simulink model "RPEM"  (Simulink 5.0)
settings: Solver=ode45  StartTime=0.0  StopTime=100.0  RelTol=1e-3
undefined symbols (not defined in the file): ts
libraries: dspmtrx3 x6, simulink x4, dspinverses x1
settings Model: LastModifiedBy=LeO

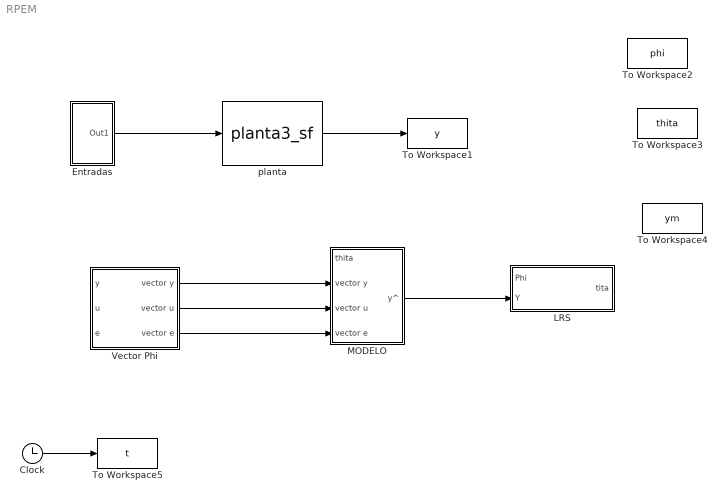
== system RPEM ==
  Clock : Clock
      settings: Decimation=10
  Entradas : Subsystem
  LRS : Subsystem
  MODELO : Subsystem
  To Workspace1 : ToWorkspace  VariableName=y  SampleTime=ts  SaveFormat=Array
  To Workspace2 : ToWorkspace  VariableName=phi  SampleTime=ts  SaveFormat=Array
  To Workspace3 : ToWorkspace  VariableName=thita  SampleTime=ts  SaveFormat=Array
  To Workspace4 : ToWorkspace  VariableName=ym  SampleTime=ts  SaveFormat=Array
  To Workspace5 : ToWorkspace  VariableName=t  SampleTime=ts  SaveFormat=Array
  Vector Phi : Subsystem  mask{nu=1, ny=3, ne=1, nk=1}
      mask prompts: nu "Nº de u tomadas"; ny "Nº de y tomadas"; ne "Nº de e tomadas"; nk "Nº de retardo"
  planta : S-Function  FunctionName=planta3_sf
  wires:
  Entradas/1(Out1) -> planta/1
  planta/1 -> To Workspace1/1
  Clock/1 -> To Workspace5/1
  MODELO/1(y^) -> LRS/2(Y)
  Vector Phi/1(vector y) -> MODELO/2(vector y)
  Vector Phi/2(vector u) -> MODELO/3(vector u)
  Vector Phi/3(vector e) -> MODELO/4("vector e ")

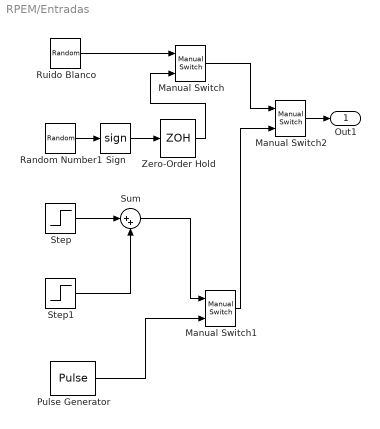
== system RPEM/Entradas ==
  Manual Switch : simulink/Signal Routing/Manual Switch  sw=0  action=0
  Manual Switch1 : simulink/Signal Routing/Manual Switch  sw=1  action=0
  Manual Switch2 : simulink/Signal Routing/Manual Switch  sw=0  action=0
  Pulse Generator : DiscretePulseGenerator  PulseType=Time based  PulseWidth=50
  Random Number1 : RandomNumber  SampleTime=0
  Ruido Blanco : RandomNumber  Variance=20  Seed=12  SampleTime=ts
  Sign : Signum
  Step : Step  Time=10  After=25  SampleTime=0.05
  Step1 : Step  Time=30  After=3  SampleTime=0.05
  Sum : Sum  Inputs=|++  SaturateOnIntegerOverflow=on
  Zero-Order Hold : ZeroOrderHold  SampleTime=0.05
  Out1 : Outport
  wires:
  Sign/1 -> Zero-Order Hold/1
  Random Number1/1 -> Sign/1
  Manual Switch/1 -> Manual Switch2/1
  Ruido Blanco/1 -> Manual Switch/1
  Zero-Order Hold/1 -> Manual Switch/2
  Manual Switch2/1 -> Out1/1
  Step/1 -> Sum/1
  Step1/1 -> Sum/2
  Manual Switch1/1 -> Manual Switch2/2
  Sum/1 -> Manual Switch1/1
  Pulse Generator/1 -> Manual Switch1/2

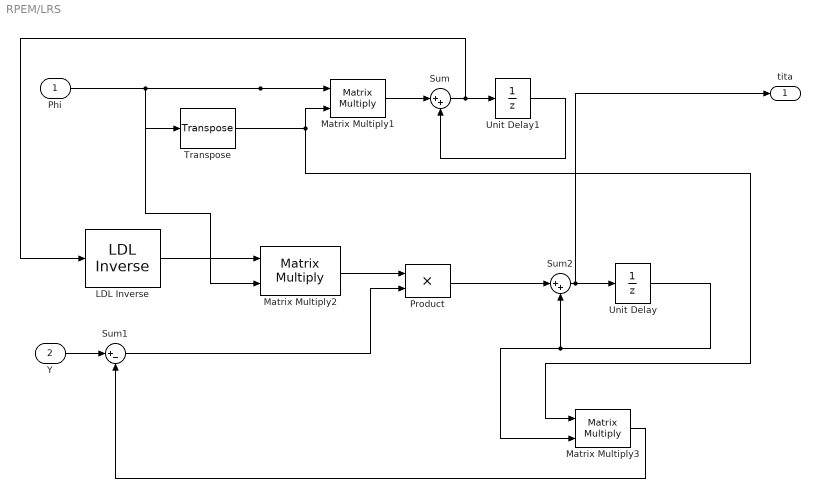
== system RPEM/LRS ==
  "Phi " : Inport  SampleTime=ts
  Y : Inport  Port=2  SampleTime=ts
  LDL Inverse : dspinverses/LDL Inverse  errmode=Ignore
  Matrix Multiply1 : dspmtrx3/Matrix Multiply  numInputPorts=2  OptimizationLevel=None
  Matrix Multiply2 : dspmtrx3/Matrix Multiply  numInputPorts=2  OptimizationLevel=None
  Matrix Multiply3 : dspmtrx3/Matrix Multiply  numInputPorts=2  OptimizationLevel=None
  Product : Product  SaturateOnIntegerOverflow=on
  Sum : Sum  Inputs=|++  SaturateOnIntegerOverflow=on
  Sum1 : Sum  Inputs=|+-  SaturateOnIntegerOverflow=on
  Sum2 : Sum  Inputs=|++  SaturateOnIntegerOverflow=on
  Transpose : dspmtrx3/Transpose  Hermitian=off
  Unit Delay : UnitDelay  X0=1*10^-3  SampleTime=ts
  Unit Delay1 : UnitDelay  X0=10^-3  SampleTime=ts
  tita : Outport
  wires:
  "Phi "/1 -> Transpose/1, Matrix Multiply2/2, Matrix Multiply1/1
  Transpose/1 -> Matrix Multiply3/1, Matrix Multiply1/2
  Matrix Multiply1/1 -> Sum/1
  Sum/1 -> Unit Delay1/1, LDL Inverse/1
  Unit Delay1/1 -> Sum/2
  LDL Inverse/1 -> Matrix Multiply2/1
  Sum2/1 -> Unit Delay/1, tita/1
  Y/1 -> Sum1/1
  Matrix Multiply2/1 -> Product/1
  Product/1 -> Sum2/1
  Matrix Multiply3/1 -> Sum1/2
  Sum1/1 -> Product/2
  Unit Delay/1 -> Matrix Multiply3/2, Sum2/2

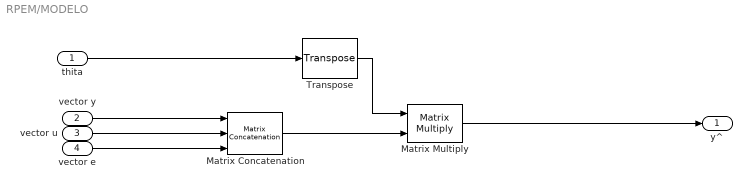
== system RPEM/MODELO ==
  thita : Inport
  vector y : Inport  Port=2
  vector u : Inport  Port=3
  "vector e " : Inport  Port=4
  Matrix Concatenation : simulink/Math Operations/Matrix Concatenation  numInports=3  catMethod=Vertical
  Matrix Multiply : dspmtrx3/Matrix Multiply  numInputPorts=2  OptimizationLevel=None
  Transpose : dspmtrx3/Transpose  Hermitian=off
  y^ : Outport
  wires:
  Matrix Concatenation/1 -> Matrix Multiply/2
  Transpose/1 -> Matrix Multiply/1
  thita/1 -> Transpose/1
  Matrix Multiply/1 -> y^/1
  "vector e "/1 -> Matrix Concatenation/3
  vector u/1 -> Matrix Concatenation/2
  vector y/1 -> Matrix Concatenation/1

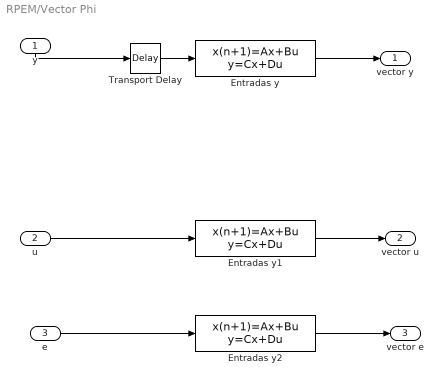
== system RPEM/Vector Phi ==
  "y " : Inport  Orientation=down  SampleTime=ts
  u : Inport  Port=2  SampleTime=ts
  e : Inport  Port=3  SampleTime=ts
  Entradas y : DiscreteStateSpace  A=[zeros(1,ny) ;eye(ny-1,ny)]  B=[[-1 zeros(1,ny-1)]']  C=[eye(ny)]  D=[zeros(1,ny)']  SampleTime=ts
  Entradas y1 : DiscreteStateSpace  A=[zeros(1,nu) ;eye(nu-1,nu)]  B=[[-1 zeros(1,nu-1)]']  C=[eye(nu)]  D=[zeros(1,nu)']  SampleTime=ts
  Entradas y2 : DiscreteStateSpace  A=[zeros(1,ne) ;eye(nu-1,ne)]  B=[[-1 zeros(1,ne-1)]']  C=[eye(ne)]  D=[zeros(1,ne)']  SampleTime=ts
  Transport Delay : TransportDelay  DelayTime=nk*ts
  vector y : Outport
  vector u : Outport  Port=2
  vector e : Outport  Port=3
  wires:
  "y "/1 -> Transport Delay/1
  u/1 -> Entradas y1/1
  Entradas y/1 -> vector y/1
  Entradas y1/1 -> vector u/1
  Transport Delay/1 -> Entradas y/1
  e/1 -> Entradas y2/1
  Entradas y2/1 -> vector e/1
